simulink model "fm"  (R2022a)
settings: Solver=VariableStepAuto  StartTime=0.0  StopTime=10.0  RelTol=1e-3
libraries: commanabbnd3 x2
settings Model: Creator=danie  LastModifiedBy=danie

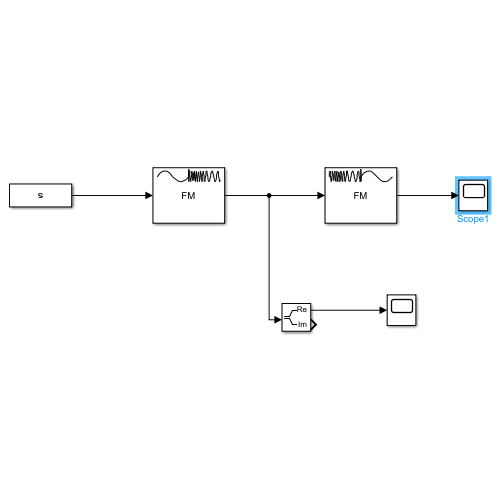
[thumbnail: Simulink's stored preview of the top-level diagram]
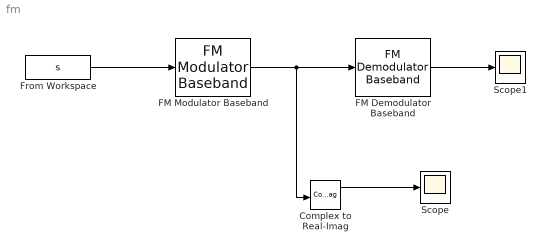
== system fm ==
  Complex to Real-Imag : ComplexToRealImag
  "FM Demodulator Baseband " : commanabbnd3/FM Demodulator Baseband   FrequencyDeviation=75e3  SimulateUsing=Code generation
      settings: SourceProductBaseCode=CM
  FM Modulator Baseband : commanabbnd3/FM Modulator Baseband  FrequencyDeviation=75e3  SimulateUsing=Code generation
      settings: SourceProductBaseCode=CM
  From Workspace : FromWorkspace  VariableName=s
  Scope : Scope
  Scope1 : Scope
  wires:
  FM Modulator Baseband/1 -> Complex to Real-Imag/1, "FM Demodulator Baseband "/1
  From Workspace/1 -> FM Modulator Baseband/1
  Complex to Real-Imag/1 -> Scope/1
  "FM Demodulator Baseband "/1 -> Scope1/1
